simulink model "ESM_TeslaModelS_statKreisfahrt"  (R2020b)
settings: Solver=FixedStepAuto  StartTime=0.0  StopTime=StopTime  FixedStep=SampleTime  RelTol=1e-3
undefined symbols (not defined in the file): ayObs, c_alpha_F, c_alpha_R, c_alpha_rear_mean, DiscIntNeverNeededParam, I_S, init, input_r, m_vehicle, par_TIR, par_VEH, parameter, SelectManeuver, simtime, Single_Track_Model_linear, SingleTrackModel_linear
libraries: pid_lib x5, simulink x3, dspsigops x2, vehicle_model x1
(part 2 of 4)

== system ESM_TeslaModelS_statKreisfahrt/Driver and Environment/BUS IN ==
  BUS_In : Inport
  Bus Selector : BusSelector  OutputSignals=Bus_Old.Dynamics.x;y;zPositionCenterofGravityandDerivates [Bus].v,Data Import.Traget_Velocity [m/s],Bus_Old.Dynamics.x;y;zPositionCenterofGravityandDerivates [Bus].y.ay [m/s^2],Data Import.Target_Radius [m],Bus_Old.Dynamics.x;y;zPositionCenterofGravityandDerivates [Bus].x.vx [m/s],Data Import.Target_Steering_Angle [rad]
  BUS : Outport  VectorParamsAs1DForOutWhenUnconnected=off
  v : Outport  Port=2  VectorParamsAs1DForOutWhenUnconnected=off
  Traget_Velocity [m/s] : Outport  Port=3  VectorParamsAs1DForOutWhenUnconnected=off
  ay [m/s^2] : Outport  Port=4  VectorParamsAs1DForOutWhenUnconnected=off
  Target_Radius [m] : Outport  Port=5  VectorParamsAs1DForOutWhenUnconnected=off
  vx [m/s] : Outport  Port=6  VectorParamsAs1DForOutWhenUnconnected=off
  Target_Steering_Angle [rad] : Outport  Port=7  VectorParamsAs1DForOutWhenUnconnected=off
  wires:
  BUS_In/1 -> BUS/1, Bus Selector/1
  Bus Selector/1 -> v/1  "<v>"
  Bus Selector/2 -> Traget_Velocity [m/s]/1  "<Traget_Velocity [m/s]>"
  Bus Selector/3 -> ay [m/s^2]/1  "<ay [m/s^2]>"
  Bus Selector/4 -> Target_Radius [m]/1  "<Target_Radius [m]>"
  Bus Selector/5 -> vx [m/s]/1  "<vx [m/s]>"
  Bus Selector/6 -> Target_Steering_Angle [rad]/1  "<Target_Steering_Angle [rad]>"

== system ESM_TeslaModelS_statKreisfahrt/Driver and Environment/BUS OUT ==
  BUS : Inport
  In1 : Inport  Port=2
  In2 : Inport  Port=3
  In3 : Inport  Port=4
  Bus Creator : BusCreator  Inputs=3
  Bus Creator1 : BusCreator  Inputs=2
  Bus Selector : BusSelector  OutputSignals=Driver and Environment,BUS.Data Import,BUS.Bus_Old  OutputAsBus=on
  BUS_OUT : Outport  VectorParamsAs1DForOutWhenUnconnected=off
  wires:
  Bus Selector/1 -> BUS_OUT/1
  Bus Creator/1 -> Bus Creator1/2  "Driver and Environment"
  BUS/1 -> Bus Creator1/1  "BUS"
  Bus Creator1/1 -> Bus Selector/1
  In1/1 -> Bus Creator/1  "delta_h"
  In2/1 -> Bus Creator/2  "AccPedalPos [-]"
  In3/1 -> Bus Creator/3  "BrakePedalPos [-]"

== system ESM_TeslaModelS_statKreisfahrt/Driver and Environment/Lenkradwinkelsprung ==
  note: Aus Library, Link wegen unterschiedlicher P und I Werte innnerhalb dieses Modells deaktiviert
  Velocity [m/s] : Inport
  TargetVelocity [m/s] : Inport  Port=2
  Driver PI Simulink_mitLenkwinkelsprung : Subsystem
  Gain : Gain  Gain=pi/180
  Ramp : simulink/Sources/Ramp  slope=15  start=simtime*0.375  InitialOutput=0.2
  Saturation : Saturate  UpperLimit=3  LowerLimit=-3
  delta_h : Outport  VectorParamsAs1DForOutWhenUnconnected=off
  AccPedalPos [-] : Outport  Port=2  VectorParamsAs1DForOutWhenUnconnected=off
  BrakePedalPos [-] : Outport  Port=3  VectorParamsAs1DForOutWhenUnconnected=off
  wires:
  Ramp/1 -> Saturation/1
  Gain/1 -> delta_h/1
  Saturation/1 -> Gain/1
  TargetVelocity [m/s]/1 -> Driver PI Simulink_mitLenkwinkelsprung/1(TargetSpd [m/s])
  Velocity [m/s]/1 -> Driver PI Simulink_mitLenkwinkelsprung/2(ActualSpeed [m/s])
  Driver PI Simulink_mitLenkwinkelsprung/2(BrakePedalPos [-]) -> BrakePedalPos [-]/1
  Driver PI Simulink_mitLenkwinkelsprung/1(AccPedalPos [-]) -> AccPedalPos [-]/1

== system ESM_TeslaModelS_statKreisfahrt/Driver and Environment/Sinuslenken ==
  note: Aus Library, Link wegen unterschiedlicher P und I Werte innnerhalb dieses Modells deaktiviert
  Velocity [m/s] : Inport
  TargetVelocity [m/s] : Inport  Port=2
  Target_Steering_Angle [rad] : Inport  Port=3
  Driver PI Simulink : Subsystem
  delta_h : Outport  VectorParamsAs1DForOutWhenUnconnected=off
  AccPedalPos [-] : Outport  Port=2  VectorParamsAs1DForOutWhenUnconnected=off
  BrakePedalPos [-] : Outport  Port=3  VectorParamsAs1DForOutWhenUnconnected=off
  wires:
  Velocity [m/s]/1 -> Driver PI Simulink/2(ActualSpeed [m/s])
  Driver PI Simulink/1(AccPedalPos [-]) -> AccPedalPos [-]/1
  TargetVelocity [m/s]/1 -> Driver PI Simulink/1(TargetSpd [m/s])
  Driver PI Simulink/2(BrakePedalPos [-]) -> BrakePedalPos [-]/1
  Target_Steering_Angle [rad]/1 -> delta_h/1

== system ESM_TeslaModelS_statKreisfahrt/Driver and Environment/quasistationare Kreisfahrt ==
  Velocity [m/s] : Inport
  TargetVelocity [m/s] : Inport  Port=2
  AccelerationY [m/s] : Inport  Port=3
  TargetRadius [m] : Inport  Port=4
  VelocityX [m/s] : Inport  Port=5
  Driver PI Simulink1 : Subsystem
  PID Driver Steering r : Subsystem  mask(SB){P_S=0, I_S=I_S, activate_stop=off, ay_stop=15}
      mask prompts: P_S "P-Value [-]"; I_S "I-Value [-]"; activate_stop "Activate Maximal lateral Acceleration"; ay_stop "Maximal lateral Acceleration (simulation stops) [m/s^2]"
      mask help:
      | <Author> Alexander Koch based on Christian Angerer </Author>
      | <Date> 04/10/2017 </Date>
      |
      | <Description>
      | PI-Controler with the ability to stop the simulation if lateral acceleration is to high.
      | </Description>
      |
      | <Parameters>
      | P-Value [-]
      | I-Value [-]
      | Activate Maximal lateral Acceleration [-]
      | Maximal lateral Acceleration (simulation stops) [m/s^2]
      | Filter Coefficient [-]
      | </Parameters>
      |
      | <Inputs>
      | VelocityX [m/s]
      | AccelerationY [m/s^2]
      | TargetRadius [m]
      | </Inputs>
      |
      | <Outputs>
      | SteeringWheelAngle [rad]
      | </Outputs>
      mask TypeOptions P_S: driver/PI-Controller/Gain/Gain
      mask TypeOptions I_S: driver/PI-Controller/I-Glied/Gain
      mask TypeOptions ay_stop: Constant1/Value
  delta_h : Outport  VectorParamsAs1DForOutWhenUnconnected=off
  AccPedalPos [-] : Outport  Port=2  VectorParamsAs1DForOutWhenUnconnected=off
  BrakePedalPos [-] : Outport  Port=3  VectorParamsAs1DForOutWhenUnconnected=off
  wires:
  PID Driver Steering r/1(SteeringWheelAngle [rad]) -> delta_h/1
  Driver PI Simulink1/1(AccPedalPos [-]) -> AccPedalPos [-]/1
  Driver PI Simulink1/2(BrakePedalPos [-]) -> BrakePedalPos [-]/1
  Velocity [m/s]/1 -> Driver PI Simulink1/2(ActualSpeed [m/s])
  TargetVelocity [m/s]/1 -> Driver PI Simulink1/1(TargetSpd [m/s])
  AccelerationY [m/s]/1 -> PID Driver Steering r/2(AccelerationY [m/s^2])
  TargetRadius [m]/1 -> PID Driver Steering r/3(TargetRadius [m])
  VelocityX [m/s]/1 -> PID Driver Steering r/1(VelocityX [m/s])

== system ESM_TeslaModelS_statKreisfahrt/Driver and Environment/quasistationare Kreisfahrt mit Lastwechsel Beschleunigung ==
  Velocity [m/s] : Inport
  TargetVelocity [m/s] : Inport  Port=2
  AccelerationY [m/s] : Inport  Port=3
  TargetRadius [m] : Inport  Port=4
  VelocityX [m/s] : Inport  Port=5
  Driver PI Simulink : Subsystem
  PID Driver Steering r_mit Lastwechsel Beschleunigung : Subsystem  mask(SB){P_S=0, I_S=I_S, activate_stop=off, ay_stop=15}
      mask prompts: P_S "P-Value [-]"; I_S "I-Value [-]"; activate_stop "Activate Maximal lateral Acceleration"; ay_stop "Maximal lateral Acceleration (simulation stops) [m/s^2]"
      mask help:
      | <Author> Alexander Koch based on Christian Angerer </Author>
      | <Date> 04/10/2017 </Date>
      |
      | <Description>
      | PI-Controler with the ability to stop the simulation if lateral acceleration is to high.
      | </Description>
      |
      | <Parameters>
      | P-Value [-]
      | I-Value [-]
      | Activate Maximal lateral Acceleration [-]
      | Maximal lateral Acceleration (simulation stops) [m/s^2]
      | Filter Coefficient [-]
      | </Parameters>
      |
      | <Inputs>
      | VelocityX [m/s]
      | AccelerationY [m/s^2]
      | TargetRadius [m]
      | </Inputs>
      |
      | <Outputs>
      | SteeringWheelAngle [rad]
      | </Outputs>
      mask TypeOptions P_S: driver/PI-Controller/Gain/Gain
      mask TypeOptions I_S: driver/PI-Controller/I-Glied/Gain
      mask TypeOptions ay_stop: Constant1/Value
  delta_h : Outport  VectorParamsAs1DForOutWhenUnconnected=off
  AccPedalPos [-] : Outport  Port=2  VectorParamsAs1DForOutWhenUnconnected=off
  BrakePedalPos [-] : Outport  Port=3  VectorParamsAs1DForOutWhenUnconnected=off
  wires:
  Driver PI Simulink/1(AccPedalPos [-]) -> AccPedalPos [-]/1
  AccelerationY [m/s]/1 -> PID Driver Steering r_mit Lastwechsel Beschleunigung/2(AccelerationY [m/s^2])
  TargetRadius [m]/1 -> PID Driver Steering r_mit Lastwechsel Beschleunigung/3(TargetRadius [m])
  PID Driver Steering r_mit Lastwechsel Beschleunigung/1(SteeringWheelAngle [rad]) -> delta_h/1
  Driver PI Simulink/2(BrakePedalPos [-]) -> BrakePedalPos [-]/1
  TargetVelocity [m/s]/1 -> Driver PI Simulink/1(TargetSpd [m/s])
  VelocityX [m/s]/1 -> PID Driver Steering r_mit Lastwechsel Beschleunigung/1(VelocityX [m/s])
  Velocity [m/s]/1 -> Driver PI Simulink/2(ActualSpeed [m/s])

== system ESM_TeslaModelS_statKreisfahrt/Driver and Environment/quasistationare Kreisfahrt mit Lastwechsel Verzogerung ==
  Velocity [m/s] : Inport
  TargetVelocity [m/s] : Inport  Port=2
  AccelerationY [m/s] : Inport  Port=3
  TargetRadius [m] : Inport  Port=4
  VelocityX [m/s] : Inport  Port=5
  Driver PI Simulink : Subsystem
  PID Driver Steering r_mit Lastwechsel Verzogerung : Subsystem  mask(SB){P_S=0, I_S=I_S, activate_stop=off, ay_stop=15}
      mask prompts: P_S "P-Value [-]"; I_S "I-Value [-]"; activate_stop "Activate Maximal lateral Acceleration"; ay_stop "Maximal lateral Acceleration (simulation stops) [m/s^2]"
      mask help:
      | <Author> Alexander Koch based on Christian Angerer </Author>
      | <Date> 04/10/2017 </Date>
      |
      | <Description>
      | PI-Controler with the ability to stop the simulation if lateral acceleration is to high.
      | </Description>
      |
      | <Parameters>
      | P-Value [-]
      | I-Value [-]
      | Activate Maximal lateral Acceleration [-]
      | Maximal lateral Acceleration (simulation stops) [m/s^2]
      | Filter Coefficient [-]
      | </Parameters>
      |
      | <Inputs>
      | VelocityX [m/s]
      | AccelerationY [m/s^2]
      | TargetRadius [m]
      | </Inputs>
      |
      | <Outputs>
      | SteeringWheelAngle [rad]
      | </Outputs>
      mask TypeOptions P_S: driver/PI-Controller/Gain/Gain
      mask TypeOptions I_S: driver/PI-Controller/I-Glied/Gain
      mask TypeOptions ay_stop: Constant1/Value
  delta_h : Outport  VectorParamsAs1DForOutWhenUnconnected=off
  AccPedalPos [-] : Outport  Port=2  VectorParamsAs1DForOutWhenUnconnected=off
  BrakePedalPos [-] : Outport  Port=3  VectorParamsAs1DForOutWhenUnconnected=off
  wires:
  Velocity [m/s]/1 -> Driver PI Simulink/2(ActualSpeed [m/s])
  VelocityX [m/s]/1 -> PID Driver Steering r_mit Lastwechsel Verzogerung/1(VelocityX [m/s])
  TargetVelocity [m/s]/1 -> Driver PI Simulink/1(TargetSpd [m/s])
  Driver PI Simulink/2(BrakePedalPos [-]) -> BrakePedalPos [-]/1
  PID Driver Steering r_mit Lastwechsel Verzogerung/1(SteeringWheelAngle [rad]) -> delta_h/1
  TargetRadius [m]/1 -> PID Driver Steering r_mit Lastwechsel Verzogerung/3(TargetRadius [m])
  AccelerationY [m/s]/1 -> PID Driver Steering r_mit Lastwechsel Verzogerung/2(AccelerationY [m/s^2])
  Driver PI Simulink/1(AccPedalPos [-]) -> AccPedalPos [-]/1

== system ESM_TeslaModelS_statKreisfahrt/Drivetrain/Axle Drive Front ==
  GearboxEntranceTorque [Nm] : Inport  SampleTime=LocalSampleTime
  RotSpdWheel [rad/s] : Inport  Port=2  SampleTime=LocalSampleTime
  JredIn [kg/m^2] : Inport  Port=3  SampleTime=LocalSampleTime
  Eta_Achsgetriebe : Constant  Value=trq_eff
  M' = M*i*eta : Product  Inputs=***
  Product : Product  Inputs=/  RndMeth=Zero
  Switch : Switch  ZeroCross=off
  i_Achsgetriebe : Constant  Value=ratio
  n' *i = n : Product  RndMeth=Zero
  n' *i = n1 : Product  RndMeth=Zero
  WheelMotTrq [Nm] : Outport  SampleTime=GlobalSampleTime  VectorParamsAs1DForOutWhenUnconnected=off
  JredOut [kg/m^2] : Outport  Port=2  SampleTime=GlobalSampleTime  VectorParamsAs1DForOutWhenUnconnected=off
  RotSpdGearboxOut [rad/s] : Outport  Port=3  SampleTime=GlobalSampleTime  VectorParamsAs1DForOutWhenUnconnected=off
  wires:
  GearboxEntranceTorque [Nm]/1 -> M' = M*i*eta/1, Switch/2
  RotSpdWheel [rad/s]/1 -> n' *i = n/2
  i_Achsgetriebe/1 -> n' *i = n/1, n' *i = n1/1, M' = M*i*eta/3
  n' *i = n/1 -> RotSpdGearboxOut [rad/s]/1
  M' = M*i*eta/1 -> WheelMotTrq [Nm]/1
  Eta_Achsgetriebe/1 -> Product/1, Switch/1
  Product/1 -> Switch/3
  Switch/1 -> M' = M*i*eta/2
  n' *i = n1/1 -> JredOut [kg/m^2]/1
  JredIn [kg/m^2]/1 -> n' *i = n1/2

== system ESM_TeslaModelS_statKreisfahrt/Drivetrain/Axle Drive Rear ==
  GearboxEntranceTorque [Nm] : Inport  SampleTime=LocalSampleTime
  RotSpdWheel [rad/s] : Inport  Port=2  SampleTime=LocalSampleTime
  JredIn [kg/m^2] : Inport  Port=3  SampleTime=LocalSampleTime
  Eta_Achsgetriebe : Constant  Value=trq_eff
  M' = M*i*eta : Product  Inputs=***
  Product : Product  Inputs=/  RndMeth=Zero
  Switch : Switch  ZeroCross=off
  i_Achsgetriebe : Constant  Value=ratio
  n' *i = n : Product  RndMeth=Zero
  n' *i = n1 : Product  RndMeth=Zero
  WheelMotTrq [Nm] : Outport  SampleTime=GlobalSampleTime  VectorParamsAs1DForOutWhenUnconnected=off
  JredOut [kg/m^2] : Outport  Port=2  SampleTime=GlobalSampleTime  VectorParamsAs1DForOutWhenUnconnected=off
  RotSpdGearboxOut [rad/s] : Outport  Port=3  SampleTime=GlobalSampleTime  VectorParamsAs1DForOutWhenUnconnected=off
  wires:
  JredIn [kg/m^2]/1 -> n' *i = n1/2
  n' *i = n1/1 -> JredOut [kg/m^2]/1
  Switch/1 -> M' = M*i*eta/2
  Product/1 -> Switch/3
  Eta_Achsgetriebe/1 -> Switch/1, Product/1
  M' = M*i*eta/1 -> WheelMotTrq [Nm]/1
  n' *i = n/1 -> RotSpdGearboxOut [rad/s]/1
  i_Achsgetriebe/1 -> M' = M*i*eta/3, n' *i = n1/1, n' *i = n/1
  RotSpdWheel [rad/s]/1 -> n' *i = n/2
  GearboxEntranceTorque [Nm]/1 -> Switch/2, M' = M*i*eta/1

== system ESM_TeslaModelS_statKreisfahrt/Drivetrain/BUS IN ==
  BUS_In : Inport
  Bus Selector : BusSelector  OutputSignals=Control Unit.TargetDriveTrqFront [Nm],Bus_Old.Dynamics.WheelRotation/Velocity [Bus].RotationSpeedWheels.omega_F [rad/s],Control Unit.TargetDriveTrqRear [Nm],Bus_Old.Dynamics.WheelRotation/Velocity [Bus].RotationSpeedWheels.omega_R [rad/s]
  BUS : Outport  VectorParamsAs1DForOutWhenUnconnected=off
  TargetDriveTrqFront [Nm] : Outport  Port=2  VectorParamsAs1DForOutWhenUnconnected=off
  omega_F [rad/s] : Outport  Port=3
  TargetDriveTrqRear [Nm] : Outport  Port=4
  omega_R [rad/s] : Outport  Port=5
  wires:
  BUS_In/1 -> Bus Selector/1, BUS/1
  Bus Selector/1 -> TargetDriveTrqFront [Nm]/1  "<TargetDriveTrqFront [Nm]>"
  Bus Selector/2 -> omega_F [rad/s]/1  "<omega_F [rad/s]>"
  Bus Selector/3 -> TargetDriveTrqRear [Nm]/1  "<TargetDriveTrqRear [Nm]>"
  Bus Selector/4 -> omega_R [rad/s]/1  "<omega_R [rad/s]>"

== system ESM_TeslaModelS_statKreisfahrt/Drivetrain/BUS OUT ==
  BUS : Inport
  In1 : Inport  Port=2
  In2 : Inport  Port=3
  In3 : Inport  Port=4
  In4 : Inport  Port=5
  Bus Creator : BusCreator  Inputs=4
  Bus Creator1 : BusCreator  Inputs=2
  Bus Selector : BusSelector  OutputSignals=Drivetrain,BUS.Control Unit,BUS.Driver and Environment,BUS.Data Import,BUS.Bus_Old  OutputAsBus=on
  BUS_OUT : Outport  VectorParamsAs1DForOutWhenUnconnected=off
  wires:
  Bus Creator1/1 -> Bus Selector/1
  BUS/1 -> Bus Creator1/1  "BUS"
  Bus Creator/1 -> Bus Creator1/2  "Drivetrain"
  Bus Selector/1 -> BUS_OUT/1
  In1/1 -> Bus Creator/1  "WheelMotTrqFront [Nm]"
  In2/1 -> Bus Creator/2  "JredOutFront [kg/m^2]"
  In3/1 -> Bus Creator/3  "WheelMotTrqRear [Nm]"
  In4/1 -> Bus Creator/4  "JredOutRear [kg/m^2]"

== system ESM_TeslaModelS_statKreisfahrt/Drivetrain/Torque_Berechnung Front ==
  note: limit output torque
  RotSpd [rad/s] : Inport
  TargetTrq [Nm] : Inport  Port=2
  Constant : Constant  Commented=on  Value=init.Inertia
  Constant1 : Constant  Value=10
  M_Reku : Lookup_n-D  NumberOfTableDimensions=1  BreakpointsForDimension1=par_VEH.dt.em.nmaxCurve_gen_VA  Table=par_VEH.dt.em.MmaxCurve_gen_VA  ExtrapMethod=Clip  UseLastTableValue=on  InternalRulePriority=Speed  RndMeth=Simplest  InputSameDT=on
  MinMax1 : MinMax  Inputs=2
  OutputTrq [Nm] : Outport  VectorParamsAs1DForOutWhenUnconnected=off
  MomentofInertia [kg m^2] : Outport  Port=2  VectorParamsAs1DForOutWhenUnconnected=off
  wires:
  TargetTrq [Nm]/1 -> MinMax1/2
  M_Reku/1 -> MinMax1/1
  Constant1/1 -> MomentofInertia [kg m^2]/1
  RotSpd [rad/s]/1 -> M_Reku/1
  MinMax1/1 -> OutputTrq [Nm]/1

== system ESM_TeslaModelS_statKreisfahrt/Drivetrain/Torque_Berechnung Rear ==
  note: limit output torque
  RotSpd [rad/s] : Inport
  TargetTrq [Nm] : Inport  Port=2
  Constant : Constant  Commented=on  Value=init.Inertia
  Constant1 : Constant  Value=10
  M_Reku : Lookup_n-D  NumberOfTableDimensions=1  BreakpointsForDimension1=par_VEH.dt.em.nmaxCurve_gen_HA  Table=par_VEH.dt.em.MmaxCurve_gen_HA  ExtrapMethod=Clip  UseLastTableValue=on  InternalRulePriority=Speed  RndMeth=Simplest  InputSameDT=on
  MinMax1 : MinMax  Inputs=2
  OutputTrq [Nm] : Outport  VectorParamsAs1DForOutWhenUnconnected=off
  MomentofInertia [kg m^2] : Outport  Port=2  VectorParamsAs1DForOutWhenUnconnected=off
  wires:
  MinMax1/1 -> OutputTrq [Nm]/1
  RotSpd [rad/s]/1 -> M_Reku/1
  Constant1/1 -> MomentofInertia [kg m^2]/1
  M_Reku/1 -> MinMax1/1
  TargetTrq [Nm]/1 -> MinMax1/2

== system ESM_TeslaModelS_statKreisfahrt/Dynamics/BUS IN ==
  BUS_In : Inport
  Bus Selector : BusSelector  OutputSignals=Drivetrain.WheelMotTrqFront [Nm],Drivetrain.WheelMotTrqRear [Nm],Control Unit.TargetBrakeTrqFrontAxle [Nm],Control Unit.TargetBrakeTrqRearAxle [Nm],Driver and Environment.delta_h
  BUS : Outport  VectorParamsAs1DForOutWhenUnconnected=off
  WheelMotTrqFront [Nm] : Outport  Port=2  VectorParamsAs1DForOutWhenUnconnected=off
  WheelMotTrqRear [Nm] : Outport  Port=3  VectorParamsAs1DForOutWhenUnconnected=off
  TargetBrakeTrqFrontAxle [Nm] : Outport  Port=4  VectorParamsAs1DForOutWhenUnconnected=off
  TargetBrakeTrqRearAxle [Nm] : Outport  Port=5  VectorParamsAs1DForOutWhenUnconnected=off
  delta_h : Outport  Port=6
  wires:
  BUS_In/1 -> Bus Selector/1, BUS/1
  Bus Selector/1 -> WheelMotTrqFront [Nm]/1  "<WheelMotTrqFront [Nm]>"
  Bus Selector/2 -> WheelMotTrqRear [Nm]/1  "<WheelMotTrqRear [Nm]>"
  Bus Selector/3 -> TargetBrakeTrqFrontAxle [Nm]/1  "<TargetBrakeTrqFrontAxle [Nm]>"
  Bus Selector/4 -> TargetBrakeTrqRearAxle [Nm]/1  "<TargetBrakeTrqRearAxle [Nm]>"
  Bus Selector/5 -> delta_h/1  "<delta_h>"

== system ESM_TeslaModelS_statKreisfahrt/Dynamics/BUS OUT ==
  BUS : Inport
  In1 : Inport  Port=2
  In2 : Inport  Port=3
  In3 : Inport  Port=4
  In4 : Inport  Port=5
  In5 : Inport  Port=6
  In6 : Inport  Port=7
  In7 : Inport  Port=8
  In8 : Inport  Port=9
  In9 : Inport  Port=10
  In10 : Inport  Port=11
  In11 : Inport  Port=12
  Bus Creator : BusCreator  Inputs=11
  Bus Creator1 : BusCreator  Inputs=2
  Bus Selector : BusSelector  OutputSignals=Dynamics,BUS.Drivetrain,BUS.Control Unit,BUS.Driver and Environment,BUS.Data Import,BUS.Bus_Old  OutputAsBus=on
  BUS_OUT : Outport  VectorParamsAs1DForOutWhenUnconnected=off
  wires:
  Bus Creator1/1 -> Bus Selector/1
  BUS/1 -> Bus Creator1/1  "BUS"
  Bus Creator/1 -> Bus Creator1/2  "Dynamics"
  Bus Selector/1 -> BUS_OUT/1
  In1/1 -> Bus Creator/1  "WheelRotation/Velocity [Bus]"
  In2/1 -> Bus Creator/2  "WheelForces [Bus]"
  In3/1 -> Bus Creator/3  "WheelMoments [Bus]"
  In4/1 -> Bus Creator/4  "DynamicWheelRadii [Bus]"
  In5/1 -> Bus Creator/5  "StaticWheelRadii [Bus]"
  In6/1 -> Bus Creator/6  "RotationalAnglesandDerivates [Bus]"
  In7/1 -> Bus Creator/7  "x,y,zPositionCenterofGravityandDerivates [Bus]"
  In8/1 -> Bus Creator/8  "SlipAnglesWheels [Bus]"
  In9/1 -> Bus Creator/9  "SideSlipAngleandDerivate [Bus]"
  In10/1 -> Bus Creator/10  "TotalSteeringAngle [Bus]"
  In11/1 -> Bus Creator/11  "AreodynamicPowerLosses [Bus]"

== system ESM_TeslaModelS_statKreisfahrt/Dynamics/Lenkübersetzung1 ==
  note: beim nach rechts Lenken beide
      | Radwinkel negativ
  note: Rechts lenken in Messung/Kennlinien positiv,
      | in Modell umgekehrt
  delta_h : Inport
  Bus Creator : BusCreator  Inputs=4
  Constant : Constant  Value=0
  Constant1 : Constant  Value=0
  Polynomial : Polyval  Coefs=par_VEH.isteer
  Polynomial1 : Polyval  Coefs=par_VEH.isteer
  Unary Minus : UnaryMinus
  Unary Minus1 : UnaryMinus
  delta_wheel : Outport  VectorParamsAs1DForOutWhenUnconnected=off
  wires:
  Bus Creator/1 -> delta_wheel/1
  Constant/1 -> Bus Creator/3  "delta_RR"
  Constant1/1 -> Bus Creator/4  "delta_LR"
  Unary Minus1/1 -> Bus Creator/2  "delta_LF"
  delta_h/1 -> Unary Minus/1, Polynomial/1
  Polynomial/1 -> Bus Creator/1  "delta_RF"
  Unary Minus/1 -> Polynomial1/1
  Polynomial1/1 -> Unary Minus1/1

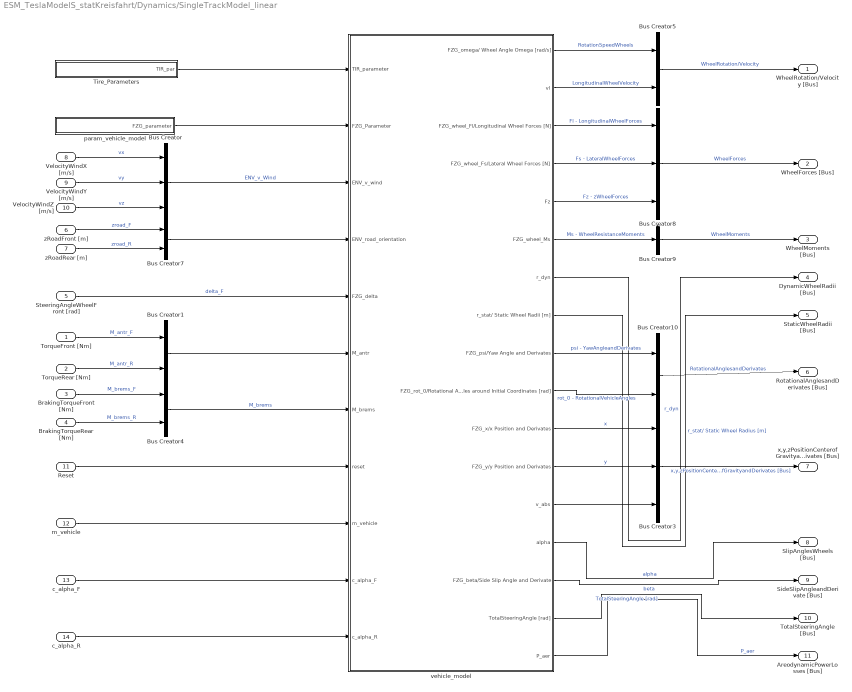
== system ESM_TeslaModelS_statKreisfahrt/Dynamics/SingleTrackModel_linear ==
  TorqueFront [Nm] : Inport
  TorqueRear [Nm] : Inport  Port=2
  BrakingTorqueFront [Nm] : Inport  Port=3
  BrakingTorqueRear [Nm] : Inport  Port=4
  SteeringAngleWheelFront [rad] : Inport  Port=5
  zRoadFront [m] : Inport  Port=6
  zRoadRear [m] : Inport  Port=7
  VelocityWindX [m/s] : Inport  Port=8
  VelocityWindY [m/s] : Inport  Port=9
  VelocityWindZ [m/s] : Inport  Port=10
  Reset : Inport  Port=11
  m_vehicle : Inport  Port=12
  c_alpha_F : Inport  Port=13
  c_alpha_R : Inport  Port=14
  Bus Creator : BusCreator  Inputs=3
  Bus Creator{1,4..5,7,10} (5 alike) : BusCreator  Inputs=2
  Bus Creator3 : BusCreator  Inputs=3
  Bus Creator8 : BusCreator  Inputs=3
  Bus Creator9 : BusCreator  Inputs=1
  Tire_Parameters : Subsystem
  param_vehicle_model : Subsystem
  vehicle_model : Subsystem  TreatAsAtomicUnit=on
      settings: MinAlgLoopOccurrences=on
  WheelRotation/Velocity [Bus] : Outport  VectorParamsAs1DForOutWhenUnconnected=off
  WheelForces [Bus] : Outport  Port=2  VectorParamsAs1DForOutWhenUnconnected=off
  WheelMoments [Bus] : Outport  Port=3  VectorParamsAs1DForOutWhenUnconnected=off
  DynamicWheelRadii [Bus] : Outport  Port=4  VectorParamsAs1DForOutWhenUnconnected=off
  StaticWheelRadii [Bus] : Outport  Port=5  VectorParamsAs1DForOutWhenUnconnected=off
  RotationalAnglesandDerivates [Bus] : Outport  Port=6  VectorParamsAs1DForOutWhenUnconnected=off
  x,y,zPositionCenterofGravityandDerivates [Bus] : Outport  Port=7  VectorParamsAs1DForOutWhenUnconnected=off
  SlipAnglesWheels [Bus] : Outport  Port=8  VectorParamsAs1DForOutWhenUnconnected=off
  SideSlipAngleandDerivate [Bus] : Outport  Port=9  VectorParamsAs1DForOutWhenUnconnected=off
  TotalSteeringAngle [Bus] : Outport  Port=10  VectorParamsAs1DForOutWhenUnconnected=off
  AreodynamicPowerLosses [Bus] : Outport  Port=11  VectorParamsAs1DForOutWhenUnconnected=off
  wires:
  Bus Creator4/1 -> vehicle_model/7(M_brems)  "M_brems"
  Bus Creator10/1 -> RotationalAnglesandDerivates [Bus]/1  "RotationalAnglesandDerivates"
  Bus Creator9/1 -> WheelMoments [Bus]/1  "WheelMoments"
  Bus Creator8/1 -> WheelForces [Bus]/1  "WheelForces"
  Bus Creator5/1 -> WheelRotation/Velocity [Bus]/1  "WheelRotation/Velocity"
  Bus Creator3/1 -> x,y,zPositionCenterofGravityandDerivates [Bus]/1  "x,y,zPositionCenterofGravityandDerivates [Bus]"
  vehicle_model/10(FZG_rot_0/Rotational Angles around Initial Coordinates [rad]) -> Bus Creator10/2  "rot_0 - RotationalVehicleAngles"
  vehicle_model/6(FZG_wheel_Ms) -> Bus Creator9/1  "Ms - WheelResistanceMoments"
  vehicle_model/4(FZG_wheel_Fs/Lateral Wheel Forces [N]) -> Bus Creator8/2  "Fs - LateralWheelForces"
  vehicle_model/15(FZG_beta/Side Slip Angle and Derivate) -> SideSlipAngleandDerivate [Bus]/1  "beta"
  vehicle_model/3(FZG_wheel_Fl/Longitudinal Wheel Forces [N]) -> Bus Creator8/1  "Fl - LongitudinalWheelForces"
  vehicle_model/12(FZG_y/y Position and Derivates) -> Bus Creator3/2  "y"
  vehicle_model/11(FZG_x/x Position and Derivates) -> Bus Creator3/1  "x"
  vehicle_model/9(FZG_psi/Yaw Angle and Derivates) -> Bus Creator10/1  "psi - YawAngleandDerivates"
  vehicle_model/1(FZG_omega/ Wheel Angle Omega [rad/s]) -> Bus Creator5/1  "RotationSpeedWheels"
  vehicle_model/7(r_dyn) -> DynamicWheelRadii [Bus]/1  "r_dyn"
  param_vehicle_model/1(FZG_parameter) -> vehicle_model/2(FZG_Parameter)
  vehicle_model/2(vl) -> Bus Creator5/2  "LongitudinalWheelVelocity"
  TorqueFront [Nm]/1 -> Bus Creator1/1  "M_antr_F"
  Tire_Parameters/1(TIR_par) -> vehicle_model/1(TIR_parameter)
  VelocityWindZ [m/s]/1 -> Bus Creator/3  "vz"
  VelocityWindY [m/s]/1 -> Bus Creator/2  "vy"
  VelocityWindX [m/s]/1 -> Bus Creator/1  "vx"
  Bus Creator/1 -> vehicle_model/3(ENV_v_wind)  "ENV_v_Wind"
  TorqueRear [Nm]/1 -> Bus Creator1/2  "M_antr_R"
  Bus Creator1/1 -> vehicle_model/6(M_antr)
  BrakingTorqueFront [Nm]/1 -> Bus Creator4/1  "M_brems_F"
  BrakingTorqueRear [Nm]/1 -> Bus Creator4/2  "M_brems_R"
  Reset/1 -> vehicle_model/8(reset)
  SteeringAngleWheelFront [rad]/1 -> vehicle_model/5(FZG_delta)  "delta_F"
  zRoadFront [m]/1 -> Bus Creator7/1  "zroad_F"
  zRoadRear [m]/1 -> Bus Creator7/2  "zroad_R"
  Bus Creator7/1 -> vehicle_model/4(ENV_road_orientation)
  vehicle_model/17(P_aer) -> AreodynamicPowerLosses [Bus]/1  "P_aer"
  vehicle_model/16(TotalSteeringAngle [rad]) -> TotalSteeringAngle [Bus]/1  "TotalSteeringAngle [rad]"
  vehicle_model/14(alpha) -> SlipAnglesWheels [Bus]/1  "alpha"
  vehicle_model/8(r_stat/ Static Wheel Radii [m]) -> StaticWheelRadii [Bus]/1  "r_stat/ Static Wheel Radius [m]"
  vehicle_model/5(Fz) -> Bus Creator8/3  "Fz - zWheelForces"
  vehicle_model/13(v_abs) -> Bus Creator3/3
  m_vehicle/1 -> vehicle_model/9(m_vehicle)
  c_alpha_F/1 -> vehicle_model/10(c_alpha_F)
  c_alpha_R/1 -> vehicle_model/11(c_alpha_R)

== system ESM_TeslaModelS_statKreisfahrt/Driver and Environment/Lenkradwinkelsprung/Driver PI Simulink_mitLenkwinkelsprung ==
  TargetSpd [m/s] : Inport
  ActualSpeed [m/s] : Inport  Port=2
  Add1 : Sum  Inputs=+-
  Constant : Constant  Value=0
  Gain5 : Gain  Gain=-1
  PID Controller : pid_lib/PID Controller  Controller=PI  Form=Parallel  TimeDomain=Discrete-time  UseExternalTs=off  SampleTime=0.05  IntegratorMethod=Forward Euler  FilterMethod=Forward Euler  ControllerParametersSource=internal  P=0.7  I=1  D=0  UseFilter=off  N=100  TunerSelectOption=Transfer Function Based (PID Tuner App)  InitialConditionSource=internal  InitialConditionForIntegrator=0  InitialConditionForFilter=0  DifferentiatorICPrevScaledInput=0  ExternalReset=level  TrackingMode=off  Kt=1  LimitOutput=on  SatLimitsSource=internal  UpperSaturationLimit=1  LowerSaturationLimit=-1  LinearizeAsGain=off  AntiWindupMode=back-calculation  Kb=1.5  POutMin=[]  POutMax=[]  IOutMin=[]  IOutMax=[]  DOutMin=[]  DOutMax=[]  NOutMin=[]  NOutMax=[]  SumOutMin=[]  SumOutMax=[]  SaturationOutMin=[]  SaturationOutMax=[]  PParamMin=[]  PParamMax=[]  IParamMin=[]  IParamMax=[]  DParamMin=[]  DParamMax=[]  NParamMin=[]  NParamMax=[]  KbParamMin=[]  KbParamMax=[]  KtParamMin=[]  KtParamMax=[]  KbOutMin=[]  KbOutMax=[]  KtOutMin=[]  KtOutMax=[]  IntegratorOutMin=[]  IntegratorOutMax=[]  FilterOutMin=[]  FilterOutMax=[]  SumI1OutMin=[]  SumI1OutMax=[]  SumI2OutMin=[]  SumI2OutMax=[]  SumI3OutMin=[]  SumI3OutMax=[]  SumI4OutMin=[]  SumI4OutMax=[]  SumDOutMin=[]  SumDOutMax=[]  DifferentiatorOutMin=[]  DifferentiatorOutMax=[]  FilterDiffOutCoefMin=[]  FilterDiffOutCoefMax=[]  ReciprocalOutMin=[]  ReciprocalOutMax=[]  SumDenOutMin=[]  SumDenOutMax=[]  SumNumOutMin=[]  SumNumOutMax=[]  DivideOutMin=[]  DivideOutMax=[]  UdiffTsProdOutMin=[]  UdiffTsProdOutMax=[]  NTsProdOutMin=[]  NTsProdOutMax=[]  UintegralTsProdOutMin=[]  UintegralTsProdOutMax=[]  UngainTsProdOutMin=[]  UngainTsProdOutMax=[]  IntegratorContinuousStateAttributes=''  IntegratorStateMustResolveToSignalObject=off  IntegratorRTWStateStorageClass=Auto  FilterContinuousStateAttributes=''  FilterStateMustResolveToSignalObject=off  FilterRTWStateStorageClass=Auto  ParallelPVariant=InternalParameters  IdealPVariant=Disabled  IVariant=InternalParameters  DVariant=Disabled  IntegratorVariant=Discrete  SatVariant=Enabled  AWVariant=BackCalculation  PCopyVariant=Disabled  TRVariant=Disabled  FdbkBlocksVariant=Forward  IdealPFdbkVariant=Disabled  SatFdbkVariant=Disabled  DerivativeFilterVariant=Disabled  NVariant=Disabled  NCopyVariant=Disabled_SignalSpec  FilterICVariant=Disabled  IntegratorICVariant=InternalICs  ExternalResetVariant=ExternalReset  TRSumVariant=Passthrough  SumFdbkVariant=Disabled  SumVariant=Sum_PI  TsampFilterVariant=InternalTs  TsampNgainVariant=Passthrough  TsampIntegralVariant=Passthrough  ExternalSaturationOutDataTypeStr=Inherit: Same as second input
  Product : Product
  Product8 : Product
  Relay : Relay  OnSwitchValue=0.02  OffSwitchValue=0
  Relay1 : Relay  OnSwitchValue=0.01  OffSwitchValue=0
  Saturation1 : Saturate  UpperLimit=1  LowerLimit=0
  Saturation2 : Saturate  UpperLimit=1  LowerLimit=0
  AccPedalPos [-] : Outport  VectorParamsAs1DForOutWhenUnconnected=off
  BrakePedalPos [-] : Outport  Port=2  VectorParamsAs1DForOutWhenUnconnected=off
  wires:
  Relay1/1 -> Product8/2
  Gain5/1 -> Saturation2/1, Relay1/1
  Relay/1 -> Product/1
  Saturation1/1 -> Product/2
  PID Controller/1 -> Gain5/1, Saturation1/1, Relay/1
  ActualSpeed [m/s]/1 -> Add1/2
  TargetSpd [m/s]/1 -> Add1/1
  Saturation2/1 -> Product8/1
  Add1/1 -> PID Controller/1
  Product8/1 -> BrakePedalPos [-]/1
  Product/1 -> AccPedalPos [-]/1
  Constant/1 -> PID Controller/2

== system ESM_TeslaModelS_statKreisfahrt/Driver and Environment/Sinuslenken/Driver PI Simulink ==
  TargetSpd [m/s] : Inport
  ActualSpeed [m/s] : Inport  Port=2
  Add1 : Sum  Inputs=+-
  Constant : Constant  Value=0
  Gain5 : Gain  Gain=-1
  PID Controller : pid_lib/PID Controller  Controller=PI  Form=Parallel  TimeDomain=Discrete-time  UseExternalTs=off  SampleTime=-1  IntegratorMethod=Forward Euler  FilterMethod=Forward Euler  ControllerParametersSource=internal  P=0.7  I=1  D=0  UseFilter=off  N=100  TunerSelectOption=Transfer Function Based (PID Tuner App)  InitialConditionSource=internal  InitialConditionForIntegrator=0  InitialConditionForFilter=0  DifferentiatorICPrevScaledInput=0  ExternalReset=level  TrackingMode=off  Kt=1  LimitOutput=on  SatLimitsSource=internal  UpperSaturationLimit=1  LowerSaturationLimit=-1  LinearizeAsGain=off  AntiWindupMode=back-calculation  Kb=1.5  POutMin=[]  POutMax=[]  IOutMin=[]  IOutMax=[]  DOutMin=[]  DOutMax=[]  NOutMin=[]  NOutMax=[]  SumOutMin=[]  SumOutMax=[]  SaturationOutMin=[]  SaturationOutMax=[]  PParamMin=[]  PParamMax=[]  IParamMin=[]  IParamMax=[]  DParamMin=[]  DParamMax=[]  NParamMin=[]  NParamMax=[]  KbParamMin=[]  KbParamMax=[]  KtParamMin=[]  KtParamMax=[]  KbOutMin=[]  KbOutMax=[]  KtOutMin=[]  KtOutMax=[]  IntegratorOutMin=[]  IntegratorOutMax=[]  FilterOutMin=[]  FilterOutMax=[]  SumI1OutMin=[]  SumI1OutMax=[]  SumI2OutMin=[]  SumI2OutMax=[]  SumI3OutMin=[]  SumI3OutMax=[]  SumI4OutMin=[]  SumI4OutMax=[]  SumDOutMin=[]  SumDOutMax=[]  DifferentiatorOutMin=[]  DifferentiatorOutMax=[]  FilterDiffOutCoefMin=[]  FilterDiffOutCoefMax=[]  ReciprocalOutMin=[]  ReciprocalOutMax=[]  SumDenOutMin=[]  SumDenOutMax=[]  SumNumOutMin=[]  SumNumOutMax=[]  DivideOutMin=[]  DivideOutMax=[]  UdiffTsProdOutMin=[]  UdiffTsProdOutMax=[]  NTsProdOutMin=[]  NTsProdOutMax=[]  UintegralTsProdOutMin=[]  UintegralTsProdOutMax=[]  UngainTsProdOutMin=[]  UngainTsProdOutMax=[]  IntegratorContinuousStateAttributes=''  IntegratorStateMustResolveToSignalObject=off  IntegratorRTWStateStorageClass=Auto  FilterContinuousStateAttributes=''  FilterStateMustResolveToSignalObject=off  FilterRTWStateStorageClass=Auto  ParallelPVariant=InternalParameters  IdealPVariant=Disabled  IVariant=InternalParameters  DVariant=Disabled  IntegratorVariant=Discrete  SatVariant=Enabled  AWVariant=BackCalculation  PCopyVariant=Disabled  TRVariant=Disabled  FdbkBlocksVariant=Forward  IdealPFdbkVariant=Disabled  SatFdbkVariant=Disabled  DerivativeFilterVariant=Disabled  NVariant=Disabled  NCopyVariant=Disabled_SignalSpec  FilterICVariant=Disabled  IntegratorICVariant=InternalICs  ExternalResetVariant=ExternalReset  TRSumVariant=Passthrough  SumFdbkVariant=Disabled  SumVariant=Sum_PI  TsampFilterVariant=InternalTs  TsampNgainVariant=Passthrough  TsampIntegralVariant=Passthrough  ExternalSaturationOutDataTypeStr=Inherit: Same as second input
  Product : Product
  Product8 : Product
  Relay : Relay  OnSwitchValue=0.02  OffSwitchValue=0
  Relay1 : Relay  OnSwitchValue=0.01  OffSwitchValue=0
  Saturation1 : Saturate  UpperLimit=1  LowerLimit=0
  Saturation2 : Saturate  UpperLimit=1  LowerLimit=0
  AccPedalPos [-] : Outport  VectorParamsAs1DForOutWhenUnconnected=off
  BrakePedalPos [-] : Outport  Port=2  VectorParamsAs1DForOutWhenUnconnected=off
  wires:
  Relay1/1 -> Product8/2
  Gain5/1 -> Saturation2/1, Relay1/1
  Relay/1 -> Product/1
  Saturation1/1 -> Product/2
  PID Controller/1 -> Gain5/1, Saturation1/1, Relay/1
  ActualSpeed [m/s]/1 -> Add1/2
  TargetSpd [m/s]/1 -> Add1/1
  Saturation2/1 -> Product8/1
  Add1/1 -> PID Controller/1
  Product8/1 -> BrakePedalPos [-]/1
  Product/1 -> AccPedalPos [-]/1
  Constant/1 -> PID Controller/2

== system ESM_TeslaModelS_statKreisfahrt/Driver and Environment/quasistationare Kreisfahrt/Driver PI Simulink1 ==
  TargetSpd [m/s] : Inport
  ActualSpeed [m/s] : Inport  Port=2
  Add1 : Sum  Inputs=+-
  Constant : Constant  Value=0
  Gain5 : Gain  Gain=-1
  PID Controller : pid_lib/PID Controller  Controller=PI  Form=Parallel  TimeDomain=Discrete-time  UseExternalTs=off  SampleTime=-1  IntegratorMethod=Forward Euler  FilterMethod=Forward Euler  ControllerParametersSource=internal  P=1.6  I=0.6  D=0  UseFilter=off  N=100  TunerSelectOption=Transfer Function Based (PID Tuner App)  InitialConditionSource=internal  InitialConditionForIntegrator=0  InitialConditionForFilter=0  DifferentiatorICPrevScaledInput=0  ExternalReset=level  TrackingMode=off  Kt=1  LimitOutput=on  SatLimitsSource=internal  UpperSaturationLimit=1  LowerSaturationLimit=-1  LinearizeAsGain=off  AntiWindupMode=back-calculation  Kb=1.5  POutMin=[]  POutMax=[]  IOutMin=[]  IOutMax=[]  DOutMin=[]  DOutMax=[]  NOutMin=[]  NOutMax=[]  SumOutMin=[]  SumOutMax=[]  SaturationOutMin=[]  SaturationOutMax=[]  PParamMin=[]  PParamMax=[]  IParamMin=[]  IParamMax=[]  DParamMin=[]  DParamMax=[]  NParamMin=[]  NParamMax=[]  KbParamMin=[]  KbParamMax=[]  KtParamMin=[]  KtParamMax=[]  KbOutMin=[]  KbOutMax=[]  KtOutMin=[]  KtOutMax=[]  IntegratorOutMin=[]  IntegratorOutMax=[]  FilterOutMin=[]  FilterOutMax=[]  SumI1OutMin=[]  SumI1OutMax=[]  SumI2OutMin=[]  SumI2OutMax=[]  SumI3OutMin=[]  SumI3OutMax=[]  SumI4OutMin=[]  SumI4OutMax=[]  SumDOutMin=[]  SumDOutMax=[]  DifferentiatorOutMin=[]  DifferentiatorOutMax=[]  FilterDiffOutCoefMin=[]  FilterDiffOutCoefMax=[]  ReciprocalOutMin=[]  ReciprocalOutMax=[]  SumDenOutMin=[]  SumDenOutMax=[]  SumNumOutMin=[]  SumNumOutMax=[]  DivideOutMin=[]  DivideOutMax=[]  UdiffTsProdOutMin=[]  UdiffTsProdOutMax=[]  NTsProdOutMin=[]  NTsProdOutMax=[]  UintegralTsProdOutMin=[]  UintegralTsProdOutMax=[]  UngainTsProdOutMin=[]  UngainTsProdOutMax=[]  IntegratorContinuousStateAttributes=''  IntegratorStateMustResolveToSignalObject=off  IntegratorRTWStateStorageClass=Auto  FilterContinuousStateAttributes=''  FilterStateMustResolveToSignalObject=off  FilterRTWStateStorageClass=Auto  ParallelPVariant=InternalParameters  IdealPVariant=Disabled  IVariant=InternalParameters  DVariant=Disabled  IntegratorVariant=Discrete  SatVariant=Enabled  AWVariant=BackCalculation  PCopyVariant=Disabled  TRVariant=Disabled  FdbkBlocksVariant=Forward  IdealPFdbkVariant=Disabled  SatFdbkVariant=Disabled  DerivativeFilterVariant=Disabled  NVariant=Disabled  NCopyVariant=Disabled_SignalSpec  FilterICVariant=Disabled  IntegratorICVariant=InternalICs  ExternalResetVariant=ExternalReset  TRSumVariant=Passthrough  SumFdbkVariant=Disabled  SumVariant=Sum_PI  TsampFilterVariant=InternalTs  TsampNgainVariant=Passthrough  TsampIntegralVariant=Passthrough  ExternalSaturationOutDataTypeStr=Inherit: Same as second input
  Product : Product
  Product8 : Product
  Relay : Relay  OnSwitchValue=0.02  OffSwitchValue=0
  Relay1 : Relay  OnSwitchValue=0.01  OffSwitchValue=0
  Saturation1 : Saturate  UpperLimit=1  LowerLimit=0
  Saturation2 : Saturate  UpperLimit=1  LowerLimit=0
  AccPedalPos [-] : Outport  VectorParamsAs1DForOutWhenUnconnected=off
  BrakePedalPos [-] : Outport  Port=2  VectorParamsAs1DForOutWhenUnconnected=off
  wires:
  Relay1/1 -> Product8/2
  Gain5/1 -> Saturation2/1, Relay1/1
  Relay/1 -> Product/1
  Saturation1/1 -> Product/2
  PID Controller/1 -> Saturation1/1, Relay/1, Gain5/1
  ActualSpeed [m/s]/1 -> Add1/2
  TargetSpd [m/s]/1 -> Add1/1
  Saturation2/1 -> Product8/1
  Add1/1 -> PID Controller/1
  Product8/1 -> BrakePedalPos [-]/1  "BrakePedalPos [-]"
  Product/1 -> AccPedalPos [-]/1  "AccPedalPos [-]"
  Constant/1 -> PID Controller/2

== system ESM_TeslaModelS_statKreisfahrt/Driver and Environment/quasistationare Kreisfahrt/PID Driver Steering r ==
  note: driver 2
  VelocityX [m/s] : Inport
  AccelerationY [m/s^2] : Inport  Port=2
  TargetRadius [m] : Inport  Port=3
  Abs : Abs
  Constant1 : Constant  Value=ay_stop
  Constant2 : Constant  Value=activate_stop
  Constant3 : Constant  Value=0
  Divide : Product  Inputs=*/
  Math Function : Math  Operator=square  SignedPower=on  SaturateOnIntegerOverflow=on
  Stop Simulation : Stop
  Subtract : Sum  Inputs=+-
  Switch : Switch  Criteria=u2 > Threshold
  driver : Subsystem
  not_zero : Subsystem
  SteeringWheelAngle [rad] : Outport  VectorParamsAs1DForOutWhenUnconnected=off
  wires:
  Switch/1 -> Stop Simulation/1
  VelocityX [m/s]/1 -> Math Function/1
  not_zero/1(Out1) -> Divide/2
  Abs/1 -> Subtract/1
  Subtract/1 -> Switch/2
  Constant1/1 -> Subtract/2
  Math Function/1 -> Divide/1
  AccelerationY [m/s^2]/1 -> Abs/1, not_zero/1(In1)
  TargetRadius [m]/1 -> driver/2(r soll)
  Constant3/1 -> Switch/3
  driver/1(delta_h) -> SteeringWheelAngle [rad]/1  "delta_h"
  Constant2/1 -> Switch/1
  Divide/1 -> driver/1(r ist)  "r_ist"

== system ESM_TeslaModelS_statKreisfahrt/Driver and Environment/quasistationare Kreisfahrt mit Lastwechsel Beschleunigung/Driver PI Simulink ==
  TargetSpd [m/s] : Inport
  ActualSpeed [m/s] : Inport  Port=2
  Add1 : Sum  Inputs=+-
  Constant : Constant  Value=0
  Gain5 : Gain  Gain=-1
  PID Controller : pid_lib/PID Controller  Controller=PI  Form=Parallel  TimeDomain=Discrete-time  UseExternalTs=off  SampleTime=-1  IntegratorMethod=Forward Euler  FilterMethod=Forward Euler  ControllerParametersSource=internal  P=1.6  I=0.6  D=0  UseFilter=off  N=100  TunerSelectOption=Transfer Function Based (PID Tuner App)  InitialConditionSource=internal  InitialConditionForIntegrator=0  InitialConditionForFilter=0  DifferentiatorICPrevScaledInput=0  ExternalReset=level  TrackingMode=off  Kt=1  LimitOutput=on  SatLimitsSource=internal  UpperSaturationLimit=1  LowerSaturationLimit=-1  LinearizeAsGain=off  AntiWindupMode=back-calculation  Kb=1.5  POutMin=[]  POutMax=[]  IOutMin=[]  IOutMax=[]  DOutMin=[]  DOutMax=[]  NOutMin=[]  NOutMax=[]  SumOutMin=[]  SumOutMax=[]  SaturationOutMin=[]  SaturationOutMax=[]  PParamMin=[]  PParamMax=[]  IParamMin=[]  IParamMax=[]  DParamMin=[]  DParamMax=[]  NParamMin=[]  NParamMax=[]  KbParamMin=[]  KbParamMax=[]  KtParamMin=[]  KtParamMax=[]  KbOutMin=[]  KbOutMax=[]  KtOutMin=[]  KtOutMax=[]  IntegratorOutMin=[]  IntegratorOutMax=[]  FilterOutMin=[]  FilterOutMax=[]  SumI1OutMin=[]  SumI1OutMax=[]  SumI2OutMin=[]  SumI2OutMax=[]  SumI3OutMin=[]  SumI3OutMax=[]  SumI4OutMin=[]  SumI4OutMax=[]  SumDOutMin=[]  SumDOutMax=[]  DifferentiatorOutMin=[]  DifferentiatorOutMax=[]  FilterDiffOutCoefMin=[]  FilterDiffOutCoefMax=[]  ReciprocalOutMin=[]  ReciprocalOutMax=[]  SumDenOutMin=[]  SumDenOutMax=[]  SumNumOutMin=[]  SumNumOutMax=[]  DivideOutMin=[]  DivideOutMax=[]  UdiffTsProdOutMin=[]  UdiffTsProdOutMax=[]  NTsProdOutMin=[]  NTsProdOutMax=[]  UintegralTsProdOutMin=[]  UintegralTsProdOutMax=[]  UngainTsProdOutMin=[]  UngainTsProdOutMax=[]  IntegratorContinuousStateAttributes=''  IntegratorStateMustResolveToSignalObject=off  IntegratorRTWStateStorageClass=Auto  FilterContinuousStateAttributes=''  FilterStateMustResolveToSignalObject=off  FilterRTWStateStorageClass=Auto  ParallelPVariant=InternalParameters  IdealPVariant=Disabled  IVariant=InternalParameters  DVariant=Disabled  IntegratorVariant=Discrete  SatVariant=Enabled  AWVariant=BackCalculation  PCopyVariant=Disabled  TRVariant=Disabled  FdbkBlocksVariant=Forward  IdealPFdbkVariant=Disabled  SatFdbkVariant=Disabled  DerivativeFilterVariant=Disabled  NVariant=Disabled  NCopyVariant=Disabled_SignalSpec  FilterICVariant=Disabled  IntegratorICVariant=InternalICs  ExternalResetVariant=ExternalReset  TRSumVariant=Passthrough  SumFdbkVariant=Disabled  SumVariant=Sum_PI  TsampFilterVariant=InternalTs  TsampNgainVariant=Passthrough  TsampIntegralVariant=Passthrough  ExternalSaturationOutDataTypeStr=Inherit: Same as second input
  Product : Product
  Product8 : Product
  Relay : Relay  OnSwitchValue=0.02  OffSwitchValue=0
  Relay1 : Relay  OnSwitchValue=0.01  OffSwitchValue=0
  Saturation1 : Saturate  UpperLimit=1  LowerLimit=0
  Saturation2 : Saturate  UpperLimit=1  LowerLimit=0
  AccPedalPos [-] : Outport  VectorParamsAs1DForOutWhenUnconnected=off
  BrakePedalPos [-] : Outport  Port=2  VectorParamsAs1DForOutWhenUnconnected=off
  wires:
  Product/1 -> AccPedalPos [-]/1  "AccPedalPos [-]"
  Product8/1 -> BrakePedalPos [-]/1  "BrakePedalPos [-]"
  Add1/1 -> PID Controller/1
  Saturation2/1 -> Product8/1
  TargetSpd [m/s]/1 -> Add1/1
  ActualSpeed [m/s]/1 -> Add1/2
  PID Controller/1 -> Relay/1, Saturation1/1, Gain5/1
  Saturation1/1 -> Product/2
  Relay/1 -> Product/1
  Gain5/1 -> Relay1/1, Saturation2/1
  Relay1/1 -> Product8/2
  Constant/1 -> PID Controller/2

== system ESM_TeslaModelS_statKreisfahrt/Driver and Environment/quasistationare Kreisfahrt mit Lastwechsel Beschleunigung/PID Driver Steering r_mit Lastwechsel Beschleunigung ==
  note: driver 2
  VelocityX [m/s] : Inport
  AccelerationY [m/s^2] : Inport  Port=2
  TargetRadius [m] : Inport  Port=3
  Abs : Abs
  Constant1 : Constant  Value=ay_stop
  Constant2 : Constant  Value=activate_stop
  Constant3 : Constant  Value=0
  Divide : Product  Inputs=*/
  Math Function : Math  Operator=square  SignedPower=on  SaturateOnIntegerOverflow=on
  Stop Simulation : Stop
  Subtract : Sum  Inputs=+-
  Switch : Switch  Criteria=u2 > Threshold
  driver : Subsystem
  not_zero : Subsystem
  SteeringWheelAngle [rad] : Outport  VectorParamsAs1DForOutWhenUnconnected=off
  wires:
  Switch/1 -> Stop Simulation/1
  Divide/1 -> driver/1(r ist)  "r_ist"
  VelocityX [m/s]/1 -> Math Function/1
  not_zero/1(Out1) -> Divide/2
  Abs/1 -> Subtract/1
  Subtract/1 -> Switch/2
  Constant1/1 -> Subtract/2
  Math Function/1 -> Divide/1
  AccelerationY [m/s^2]/1 -> Abs/1, not_zero/1(In1)
  TargetRadius [m]/1 -> driver/2(r soll)
  Constant3/1 -> Switch/3
  driver/1(delta_h) -> SteeringWheelAngle [rad]/1  "delta_h"
  Constant2/1 -> Switch/1

== system ESM_TeslaModelS_statKreisfahrt/Driver and Environment/quasistationare Kreisfahrt mit Lastwechsel Verzogerung/Driver PI Simulink ==
  TargetSpd [m/s] : Inport
  ActualSpeed [m/s] : Inport  Port=2
  Add1 : Sum  Inputs=+-
  Constant : Constant  Value=0
  Gain5 : Gain  Gain=-1
  PID Controller : pid_lib/PID Controller  Controller=PI  Form=Parallel  TimeDomain=Discrete-time  UseExternalTs=off  SampleTime=-1  IntegratorMethod=Forward Euler  FilterMethod=Forward Euler  ControllerParametersSource=internal  P=1.6  I=0.6  D=0  UseFilter=off  N=100  TunerSelectOption=Transfer Function Based (PID Tuner App)  InitialConditionSource=internal  InitialConditionForIntegrator=0  InitialConditionForFilter=0  DifferentiatorICPrevScaledInput=0  ExternalReset=level  TrackingMode=off  Kt=1  LimitOutput=on  SatLimitsSource=internal  UpperSaturationLimit=1  LowerSaturationLimit=-1  LinearizeAsGain=off  AntiWindupMode=back-calculation  Kb=1.5  POutMin=[]  POutMax=[]  IOutMin=[]  IOutMax=[]  DOutMin=[]  DOutMax=[]  NOutMin=[]  NOutMax=[]  SumOutMin=[]  SumOutMax=[]  SaturationOutMin=[]  SaturationOutMax=[]  PParamMin=[]  PParamMax=[]  IParamMin=[]  IParamMax=[]  DParamMin=[]  DParamMax=[]  NParamMin=[]  NParamMax=[]  KbParamMin=[]  KbParamMax=[]  KtParamMin=[]  KtParamMax=[]  KbOutMin=[]  KbOutMax=[]  KtOutMin=[]  KtOutMax=[]  IntegratorOutMin=[]  IntegratorOutMax=[]  FilterOutMin=[]  FilterOutMax=[]  SumI1OutMin=[]  SumI1OutMax=[]  SumI2OutMin=[]  SumI2OutMax=[]  SumI3OutMin=[]  SumI3OutMax=[]  SumI4OutMin=[]  SumI4OutMax=[]  SumDOutMin=[]  SumDOutMax=[]  DifferentiatorOutMin=[]  DifferentiatorOutMax=[]  FilterDiffOutCoefMin=[]  FilterDiffOutCoefMax=[]  ReciprocalOutMin=[]  ReciprocalOutMax=[]  SumDenOutMin=[]  SumDenOutMax=[]  SumNumOutMin=[]  SumNumOutMax=[]  DivideOutMin=[]  DivideOutMax=[]  UdiffTsProdOutMin=[]  UdiffTsProdOutMax=[]  NTsProdOutMin=[]  NTsProdOutMax=[]  UintegralTsProdOutMin=[]  UintegralTsProdOutMax=[]  UngainTsProdOutMin=[]  UngainTsProdOutMax=[]  IntegratorContinuousStateAttributes=''  IntegratorStateMustResolveToSignalObject=off  IntegratorRTWStateStorageClass=Auto  FilterContinuousStateAttributes=''  FilterStateMustResolveToSignalObject=off  FilterRTWStateStorageClass=Auto  ParallelPVariant=InternalParameters  IdealPVariant=Disabled  IVariant=InternalParameters  DVariant=Disabled  IntegratorVariant=Discrete  SatVariant=Enabled  AWVariant=BackCalculation  PCopyVariant=Disabled  TRVariant=Disabled  FdbkBlocksVariant=Forward  IdealPFdbkVariant=Disabled  SatFdbkVariant=Disabled  DerivativeFilterVariant=Disabled  NVariant=Disabled  NCopyVariant=Disabled_SignalSpec  FilterICVariant=Disabled  IntegratorICVariant=InternalICs  ExternalResetVariant=ExternalReset  TRSumVariant=Passthrough  SumFdbkVariant=Disabled  SumVariant=Sum_PI  TsampFilterVariant=InternalTs  TsampNgainVariant=Passthrough  TsampIntegralVariant=Passthrough  ExternalSaturationOutDataTypeStr=Inherit: Same as second input
  Product : Product
  Product8 : Product
  Relay : Relay  OnSwitchValue=0.02  OffSwitchValue=0
  Relay1 : Relay  OnSwitchValue=0.01  OffSwitchValue=0
  Saturation1 : Saturate  UpperLimit=1  LowerLimit=0
  Saturation2 : Saturate  UpperLimit=1  LowerLimit=0
  AccPedalPos [-] : Outport  VectorParamsAs1DForOutWhenUnconnected=off
  BrakePedalPos [-] : Outport  Port=2  VectorParamsAs1DForOutWhenUnconnected=off
  wires:
  Relay1/1 -> Product8/2
  Gain5/1 -> Saturation2/1, Relay1/1
  Relay/1 -> Product/1
  Saturation1/1 -> Product/2
  PID Controller/1 -> Saturation1/1, Relay/1, Gain5/1
  ActualSpeed [m/s]/1 -> Add1/2
  TargetSpd [m/s]/1 -> Add1/1
  Saturation2/1 -> Product8/1
  Add1/1 -> PID Controller/1
  Product8/1 -> BrakePedalPos [-]/1  "BrakePedalPos [-]"
  Product/1 -> AccPedalPos [-]/1  "AccPedalPos [-]"
  Constant/1 -> PID Controller/2

== system ESM_TeslaModelS_statKreisfahrt/Driver and Environment/quasistationare Kreisfahrt mit Lastwechsel Verzogerung/PID Driver Steering r_mit Lastwechsel Verzogerung ==
  note: driver 2
  VelocityX [m/s] : Inport
  AccelerationY [m/s^2] : Inport  Port=2
  TargetRadius [m] : Inport  Port=3
  Abs : Abs
  Constant1 : Constant  Value=ay_stop
  Constant2 : Constant  Value=activate_stop
  Constant3 : Constant  Value=0
  Divide : Product  Inputs=*/
  Math Function : Math  Operator=square  SignedPower=on  SaturateOnIntegerOverflow=on
  Stop Simulation : Stop
  Subtract : Sum  Inputs=+-
  Switch : Switch  Criteria=u2 > Threshold
  driver : Subsystem
  not_zero : Subsystem
  SteeringWheelAngle [rad] : Outport  VectorParamsAs1DForOutWhenUnconnected=off
  wires:
  Constant2/1 -> Switch/1
  driver/1(delta_h) -> SteeringWheelAngle [rad]/1  "delta_h"
  Constant3/1 -> Switch/3
  TargetRadius [m]/1 -> driver/2(r soll)
  AccelerationY [m/s^2]/1 -> not_zero/1(In1), Abs/1
  Math Function/1 -> Divide/1
  Constant1/1 -> Subtract/2
  Subtract/1 -> Switch/2
  Abs/1 -> Subtract/1
  not_zero/1(Out1) -> Divide/2
  VelocityX [m/s]/1 -> Math Function/1
  Divide/1 -> driver/1(r ist)  "r_ist"
  Switch/1 -> Stop Simulation/1

== system ESM_TeslaModelS_statKreisfahrt/Dynamics/SingleTrackModel_linear/Tire_Parameters ==
  param_tire_model : Subsystem
  TIR_par : Outport  VectorParamsAs1DForOutWhenUnconnected=off
  wires:
  param_tire_model/1(TIR_parameter) -> TIR_par/1

== system ESM_TeslaModelS_statKreisfahrt/Dynamics/SingleTrackModel_linear/param_vehicle_model ==
  Bus Creator : BusCreator  Inputs=13
  Constant : Constant  Value=par_VEH.m
  Constant1 : Constant  Value=par_VEH.cz
  Constant2 : Constant  Value=par_VEH.RohAir
  Constant23 : Constant  Value=par_VEH.lDP
  Constant24 : Constant  Value=par_VEH.lF
  Constant25 : Constant  Value=par_VEH.lR
  Constant28 : Constant  Value=par_VEH.g
  Constant31 : Constant  Value=par_VEH.cx
  Constant32 : Constant  Value=par_VEH.Afront
  Constant34 : Constant  Value=par_VEH.cy
  Constant5 : Constant  Value=par_VEH.Iz
  Constant6 : Constant  Value=par_VEH.xSP
  Constant9 : Constant  Value=par_VEH.l
  FZG_parameter : Outport  VectorParamsAs1DForOutWhenUnconnected=off
  wires:
  Constant1/1 -> Bus Creator/2  "cz"
  Constant23/1 -> Bus Creator/13  "lDP"
  Constant34/1 -> Bus Creator/12  "cy"
  Constant2/1 -> Bus Creator/11  "rhoair"
  Constant32/1 -> Bus Creator/10  "Afront"
  Constant31/1 -> Bus Creator/9  "cx"
  Bus Creator/1 -> FZG_parameter/1
  Constant/1 -> Bus Creator/1  "m"
  Constant5/1 -> Bus Creator/3  "Iz"
  Constant6/1 -> Bus Creator/4  "xSP"
  Constant9/1 -> Bus Creator/5  "l"
  Constant24/1 -> Bus Creator/6  "lF"
  Constant25/1 -> Bus Creator/7  "lR"
  Constant28/1 -> Bus Creator/8  "g"
